simulink model "Robot_diferencial"  (R2023b)
settings: Solver=VariableStepAuto  StartTime=0.0  StopTime=10.0  RelTol=1e-3
settings Model: Creator=alexo  LastModifiedBy=alexo

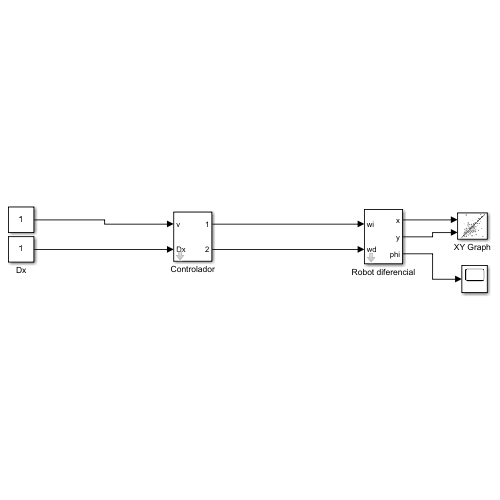
[thumbnail: Simulink's stored preview of the top-level diagram]
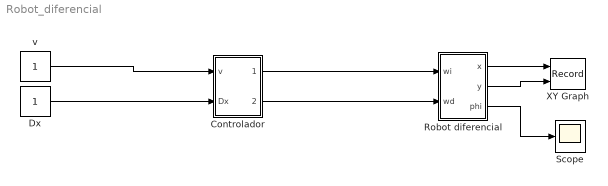
== system Robot_diferencial ==
  Controlador : Subsystem  mask{L=0, c=4, b=3}
      mask prompts: L "Distancia de seguimiento"; c "Radio de las ruedas"; b "Distancia entre las ruedas"
  Dx : Constant
  Robot diferencial : Subsystem  mask{c=4, b=3}
      mask prompts: c "Radio de las ruedas"; b "Separacion de las ruedas"
  Scope : Scope
  XY Graph : Record  FileSettingsInternal="{\"entries\":[{\"content\":{\"excelSettings\":{\"content\":{},\"type\":\"Streamout.ExcelSettings\"}},\"type\":\"Streamout.FileSettingStorage\",\"uuid\":\"\"}],\"packageUris\":[\"http:\\/\\/schema.mathworks.com\\/mf0\\/streamout_blocks\\/R2020a\"],\"version\":\"1.0\"}"  Layout=[1 1]  SignalsInternal="{\"entries\":[{\"content\":{\"signals\":[{\"content\":{\"blockPath\":[],\"dimensions\":[1],\"domain\":\"\",\"lineColor\":\"#64d413\",\"plots\":[1],\"port\":1,\"signalID\":8,\"signalName\":\"Robot diferencial:1\"},\"type\":\"RecordBlkView.Signal\",\"uuid\":\"\"},{\"content\":{\"blockPath\":[],\"dimensions\":[1],\"domain\":\"\",\"lineColor\":\"#ff13a6\",\"plots\":[1],\"port\":2,\"signalID\":11,\"signalName\":\"Robot diferencial:2\"},\"type\":\"RecordBlkView.Signal\",\"uuid\":\"\"}]},\"type\":\"RecordBlkView.InputSignals\",\"uuid\":\"\"}],\"packageUris\":[\"http:\\/\\/schema.mathworks.com\\/mf0\\/streamout_blocks\\/R2020a\"],\"version\":\"1.0\"}"  VisualizationBindings="{\"xyplotplugin\":{\"info\":[{\"series\":[{\"bindingParametersList\":[{\"parameter\":\"X-Axis\",\"signalID\":8,\"signalName\":\"Robot diferencial:1\"},{\"parameter\":\"Y-Axis\",\"signalID\":11,\"signalName\":\"Robot diferencial:2\"}],\"seriesID\":59453}],\"subplotID\":1}]}}"  CompatibilityTag=XY
  v : Constant
  wires:
  Robot diferencial/1(x) -> XY Graph/1
  Robot diferencial/2(y) -> XY Graph/2
  Robot diferencial/3(phi) -> Scope/1
  v/1 -> Controlador/1(v)
  Dx/1 -> Controlador/2(Dx)
  Controlador/1(Out1) -> Robot diferencial/1(wi)
  Controlador/2(Out2) -> Robot diferencial/2(wd)

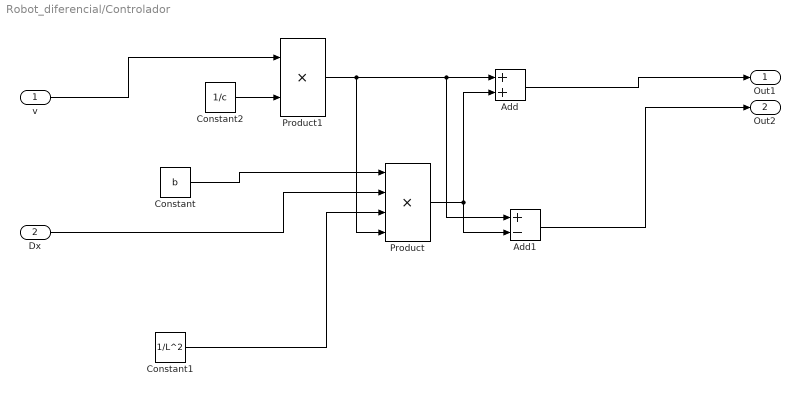
== system Robot_diferencial/Controlador ==
  v : Inport
  Dx : Inport  Port=2
  Add : Sum
  Add1 : Sum  Inputs=+-
  Constant : Constant  Value=b
  Constant1 : Constant  Value=1/L^2
  Constant2 : Constant  Value=1/c
  Product : Product  Inputs=4
  Product1 : Product
  Out1 : Outport
  Out2 : Outport  Port=2
  wires:
  Product/1 -> Add1/2, Add/2
  Product1/1 -> Add1/1, Add/1, Product/4
  Add/1 -> Out1/1
  Dx/1 -> Product/2
  Constant/1 -> Product/1
  Constant1/1 -> Product/3
  Constant2/1 -> Product1/2
  v/1 -> Product1/1
  Add1/1 -> Out2/1

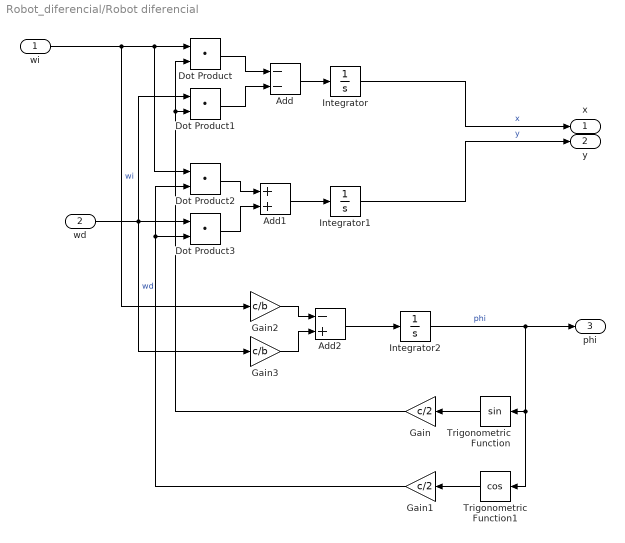
== system Robot_diferencial/Robot diferencial ==
  wi : Inport
  wd : Inport  Port=2
  Add : Sum  Inputs=--
  Add1 : Sum
  Add2 : Sum  Inputs=-+
  Dot Product{,1..3} (4 alike) : DotProduct  OutDataTypeStr=Inherit: Inherit via internal rule
  Gain : Gain  Gain=c/2
  Gain1 : Gain  Gain=c/2
  Gain2 : Gain  Gain=c/b
  Gain3 : Gain  Gain=c/b
  Integrator : Integrator
  Integrator1 : Integrator
  Integrator2 : Integrator
  Trigonometric Function : Trigonometry
  Trigonometric Function1 : Trigonometry  Operator=cos
  x : Outport
  y : Outport  Port=2
  phi : Outport  Port=3
  wires:
  Gain1/1 -> Dot Product3/2, Dot Product2/2
  wd/1 -> Gain3/1, Dot Product3/1, Dot Product1/1  "wd"
  wi/1 -> Gain2/1, Dot Product2/1, Dot Product/1  "wi"
  Integrator1/1 -> y/1  "y"
  Dot Product/1 -> Add/1
  Trigonometric Function1/1 -> Gain1/1
  Integrator2/1 -> phi/1, Trigonometric Function1/1, Trigonometric Function/1  "phi"
  Gain/1 -> Dot Product1/2, Dot Product/2
  Trigonometric Function/1 -> Gain/1
  Dot Product1/1 -> Add/2
  Add1/1 -> Integrator1/1
  Integrator/1 -> x/1  "x"
  Dot Product2/1 -> Add1/1
  Dot Product3/1 -> Add1/2
  Add/1 -> Integrator/1
  Gain2/1 -> Add2/1
  Add2/1 -> Integrator2/1
  Gain3/1 -> Add2/2
